simulink model "Disturbance_models"  (R2022a)
settings: Solver=VariableStepAuto  StartTime=0.0  StopTime=10.0  RelTol=1e-3
values from neighbouring files (symbols this model uses):
  A = [0 0 1 0 0 ... (first row only)    [DesignProjectP2.m]    (also in DesignProjectP3.m; DesignProject_OffsetP3.m; mpc_example_regulation.m = [ 	 0,       0,              1,  0, 0; 	 0,       0,        ; mpc_example_tracking.m = [ 	 0,       0,              1,  0, 0; 	 0,       0,        )
  A_dist = [A zeros(5,2) ... (first row only)    [DesignProjectP2.m]
  B = [0;0;0;0;1/La]    [DesignProjectP2.m]    (also in DesignProjectP3.m; DesignProject_OffsetP3.m; mpc_example_regulation.m = [0; 0; 0; 0; 1/La]; mpc_example_tracking.m = [0; 0; 0; 0; 1/La])
  B_dist = [B; zeros(2,1)]    [DesignProjectP2.m]
  C = [1 0 0 0 0 ... (first row only)    [DesignProjectP2.m]    (also in DesignProjectP3.m; DesignProject_OffsetP3.m; mpc_example_regulation.m; mpc_example_tracking.m)
  C_d = [1 0]    [DesignProjectP2.m]    (also in DesignProject_OffsetP3.m)
  C_dist = [0 1 0 0 0 zeros(1,2)]    [DesignProjectP2.m]
  init = [theta_m_init; theta_l_init; thetadot_m_init; thetadot_l_init; Ia_init]    [ELEN90064_Project_Parameters.m]
  K_sin = K_dist(1:5)    [DesignProjectP2.m]    (also in DesignProject_OffsetP3.m = K_dist(7:8))
  Kd_sin = K_dist(6:7)    [DesignProjectP2.m]
  L = place(A', C', observer_poles)'    [DesignProjectP2.m]    (also in DesignProjectP3.m; DesignProject_OffsetP3.m = L_t'; phase2_emc.m = place(A',C',desired_obsv_poles)')
  N_x = G_tf_den(end)/G_tf_num(end)    [DesignProjectP2.m]
  w = 2*pi*1/4    (= 1.57079632679)    [DesignProjectP2.m]    (also in DesignProject_OffsetP3.m)
undefined symbols (not defined in the file or in its folder): J_sin
settings Model: Creator=Admin  LastModifiedBy=Admin

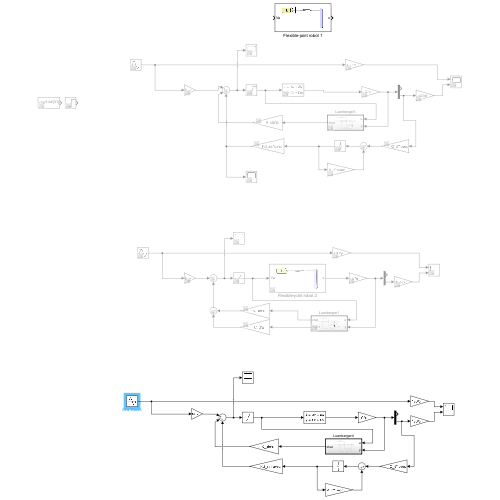
[thumbnail: Simulink's stored preview of the top-level diagram]
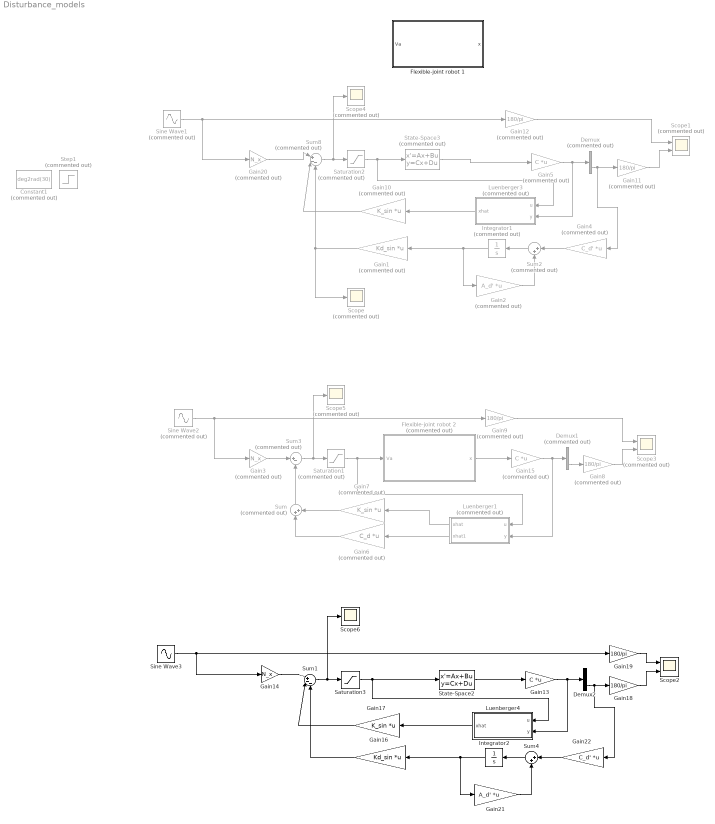
== system Disturbance_models ==
  Constant1 : Constant  Commented=on  Value=deg2rad(30)
  Demux : Demux  Commented=on  Outputs=2
  Demux1 : Demux  Commented=on  Outputs=2
  Demux2 : Demux  Outputs=2
  Flexible-joint robot 1 : Subsystem
      mask Display: image('$imagefile'); % Use "Edit Image" on toolstrip to change.
  Flexible-joint robot 2 : Subsystem  Commented=on
      mask Display: image('$imagefile'); % Use "Edit Image" on toolstrip to change.
  Gain1 : Gain  Commented=on  Gain=Kd_sin  Multiplication=Matrix(K*u) (u vector)
  Gain10 : Gain  Commented=on  Gain=K_sin  Multiplication=Matrix(K*u)
  Gain{8..9,11..12} (4 alike) : Gain  Commented=on  Gain=180/pi
  Gain13 : Gain  Gain=C  Multiplication=Matrix(K*u)
  Gain14 : Gain  Gain=N_x
  Gain15 : Gain  Commented=on  Gain=C  Multiplication=Matrix(K*u)
  Gain16 : Gain  Gain=Kd_sin  Multiplication=Matrix(K*u) (u vector)
  Gain17 : Gain  Gain=K_sin  Multiplication=Matrix(K*u)
  Gain18 : Gain  Gain=180/pi
  Gain19 : Gain  Gain=180/pi
  Gain2 : Gain  Commented=on  Gain=A_d'  Multiplication=Matrix(K*u) (u vector)
  Gain20 : Gain  Commented=on  Gain=N_x
  Gain21 : Gain  Gain=A_d'  Multiplication=Matrix(K*u) (u vector)
  Gain22 : Gain  Gain=C_d'  Multiplication=Matrix(K*u) (u vector)
  Gain3 : Gain  Commented=on  Gain=N_x
  Gain4 : Gain  Commented=on  Gain=C_d'  Multiplication=Matrix(K*u) (u vector)
  Gain5 : Gain  Commented=on  Gain=C  Multiplication=Matrix(K*u)
  Gain6 : Gain  Commented=on  Gain=C_d  Multiplication=Matrix(K*u)
  Gain7 : Gain  Commented=on  Gain=K_sin  Multiplication=Matrix(K*u)
  Integrator1 : Integrator  Commented=on
  Integrator2 : Integrator
  Luenberger1 : Subsystem  Commented=on  TreatAsAtomicUnit=on
  Luenberger3 : Subsystem  Commented=on  TreatAsAtomicUnit=on
  Luenberger4 : Subsystem  TreatAsAtomicUnit=on
  Saturation1 : Saturate  Commented=on  UpperLimit=6  LowerLimit=-6
  Saturation2 : Saturate  Commented=on  UpperLimit=6  LowerLimit=-6
  Saturation3 : Saturate  UpperLimit=6  LowerLimit=-6
  Scope : Scope  Commented=on
  Scope1 : Scope  Commented=on  NumInputPorts=2
  Scope2 : Scope  NumInputPorts=2
  Scope3 : Scope  Commented=on  NumInputPorts=2
  Scope4 : Scope  Commented=on
  Scope5 : Scope  Commented=on
  Scope6 : Scope
  Sine Wave1 : Sin  Commented=on  Amplitude=deg2rad(30)  Frequency=w  Phase=deg2rad(30)  SampleTime=0
  Sine Wave2 : Sin  Commented=on  Amplitude=deg2rad(30)  Frequency=w  Phase=deg2rad(30)  SampleTime=0
  Sine Wave3 : Sin  Amplitude=deg2rad(30)  Frequency=w  Phase=deg2rad(30)  SampleTime=0
  State-Space2 : StateSpace  A=A  B=B  C=eye(5)  D=zeros(5,1)  InitialCondition=0
  State-Space3 : StateSpace  Commented=on  A=A  B=B  C=eye(5)  D=zeros(5,1)  InitialCondition=0
  Step1 : Step  Commented=on  After=deg2rad(60)  SampleTime=0
  Sum : Sum  Commented=on  Inputs=|++
  Sum1 : Sum  Inputs=|+--
  Sum2 : Sum  Commented=on  Inputs=|++
  Sum3 : Sum  Commented=on  Inputs=|+-
  Sum4 : Sum  Inputs=|++
  Sum8 : Sum  Commented=on  Inputs=|+--
  wires:
  Gain20/1 -> Sum8/1
  Gain12/1 -> Scope1/1
  State-Space3/1 -> Gain5/1
  Gain11/1 -> Scope1/2
  Gain10/1 -> Sum8/2
  Sum8/1 -> Scope4/1, Saturation2/1
  Saturation2/1 -> State-Space3/1, Luenberger3/1(u)
  Gain1/1 -> Sum8/3, Scope/1
  Demux/2 -> Gain4/1, Gain11/1
  Sine Wave1/1 -> Gain20/1, Gain12/1
  Gain2/1 -> Sum2/2
  Gain5/1 -> Demux/1, Luenberger3/2(y)
  Sum2/1 -> Integrator1/1
  Integrator1/1 -> Gain1/1, Gain2/1
  Gain4/1 -> Sum2/1
  Gain15/1 -> Demux1/1, Luenberger1/2(y)
  Sine Wave2/1 -> Gain9/1, Gain3/1
  Demux1/2 -> Gain8/1
  Luenberger1/1(xhat) -> Gain7/1
  Saturation1/1 -> Flexible-joint robot 2/1(Va), Luenberger1/1(u)
  Sum3/1 -> Saturation1/1, Scope5/1
  Gain7/1 -> Sum/2
  Gain8/1 -> Scope3/2
  Flexible-joint robot 2/1(x) -> Gain15/1
  Gain9/1 -> Scope3/1
  Gain3/1 -> Sum3/1
  Luenberger1/2(xhat1) -> Gain6/1
  Gain6/1 -> Sum/1
  Gain16/1 -> Sum1/3
  Gain14/1 -> Sum1/1
  Gain19/1 -> Scope2/1
  State-Space2/1 -> Gain13/1
  Gain18/1 -> Scope2/2
  Gain17/1 -> Sum1/2
  Sum1/1 -> Scope6/1, Saturation3/1
  Saturation3/1 -> Luenberger4/1(u), State-Space2/1
  Luenberger4/1(xhat) -> Gain17/1
  Sine Wave3/1 -> Gain19/1, Gain14/1
  Gain13/1 -> Luenberger4/2(y), Demux2/1
  Sum/1 -> Sum3/2
  Luenberger3/1(xhat) -> Gain10/1
  Sum4/1 -> Integrator2/1
  Gain21/1 -> Sum4/2
  Gain22/1 -> Sum4/1
  Integrator2/1 -> Gain16/1, Gain21/1
  Demux2/2 -> Gain22/1, Gain18/1

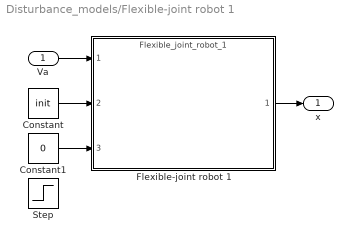
== system Disturbance_models/Flexible-joint robot 1 ==
  Va : Inport
  Constant : Constant  Value=init
  Constant1 : Constant  Value=0
  Flexible-joint robot 1 : ModelReference  ModelNameDialog=Flexible_joint_robot_1  ModelReferenceVersion=1.65  CopyOfModelProtected=on
  Step : Step  After=0.05  SampleTime=0
  x : Outport
  wires:
  Constant/1 -> Flexible-joint robot 1/2
  Flexible-joint robot 1/1 -> x/1
  Va/1 -> Flexible-joint robot 1/1
  Constant1/1 -> Flexible-joint robot 1/3

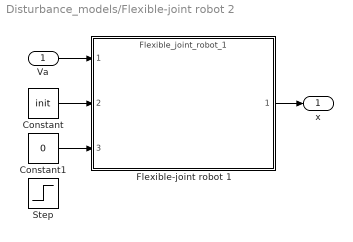
== system Disturbance_models/Flexible-joint robot 2 ==
  Va : Inport
  Constant : Constant  Value=init
  Constant1 : Constant  Value=0
  Flexible-joint robot 1 : ModelReference  ModelNameDialog=Flexible_joint_robot_1  ModelReferenceVersion=1.65  CopyOfModelProtected=on
  Step : Step  After=0.05  SampleTime=0
  x : Outport
  wires:
  Constant1/1 -> Flexible-joint robot 1/3
  Va/1 -> Flexible-joint robot 1/1
  Flexible-joint robot 1/1 -> x/1
  Constant/1 -> Flexible-joint robot 1/2

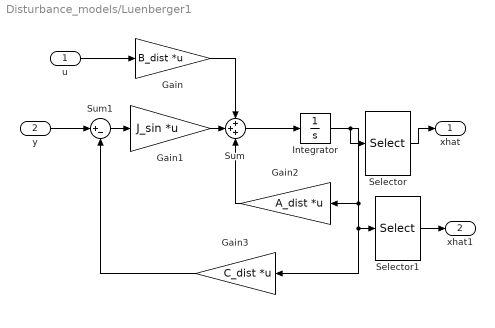
== system Disturbance_models/Luenberger1 ==
  u : Inport
  y : Inport  Port=2
  Gain : Gain  Gain=B_dist  Multiplication=Matrix(K*u) (u vector)
  Gain1 : Gain  Gain=J_sin  Multiplication=Matrix(K*u) (u vector)
  Gain2 : Gain  Gain=A_dist  Multiplication=Matrix(K*u) (u vector)
  Gain3 : Gain  Gain=C_dist  Multiplication=Matrix(K*u) (u vector)
  Integrator : Integrator
  Selector : Selector  InputPortWidth=7  IndexOptions=Index vector (dialog)  Indices=[1 2 3 4 5]  OutputSizes=1
  Selector1 : Selector  InputPortWidth=7  IndexOptions=Index vector (dialog)  Indices=[6 7]  OutputSizes=1
  Sum : Sum  Inputs=+++
  Sum1 : Sum  Inputs=|+-
  xhat : Outport
  xhat1 : Outport  Port=2
  wires:
  u/1 -> Gain/1
  Gain/1 -> Sum/1
  y/1 -> Sum1/1
  Sum1/1 -> Gain1/1
  Gain1/1 -> Sum/2
  Sum/1 -> Integrator/1
  Integrator/1 -> Selector1/1, Gain3/1, Gain2/1, Selector/1
  Gain2/1 -> Sum/3
  Gain3/1 -> Sum1/2
  Selector/1 -> xhat/1
  Selector1/1 -> xhat1/1

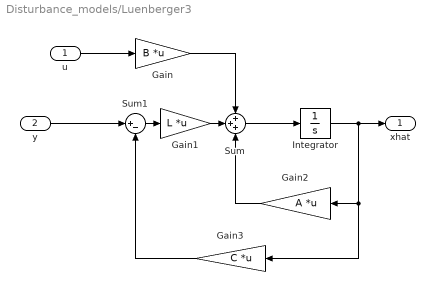
== system Disturbance_models/Luenberger3 ==
  u : Inport
  y : Inport  Port=2
  Gain : Gain  Gain=B  Multiplication=Matrix(K*u) (u vector)
  Gain1 : Gain  Gain=L  Multiplication=Matrix(K*u) (u vector)
  Gain2 : Gain  Gain=A  Multiplication=Matrix(K*u) (u vector)
  Gain3 : Gain  Gain=C  Multiplication=Matrix(K*u) (u vector)
  Integrator : Integrator
  Sum : Sum  Inputs=+++
  Sum1 : Sum  Inputs=|+-
  xhat : Outport
  wires:
  Gain3/1 -> Sum1/2
  Gain2/1 -> Sum/3
  Integrator/1 -> xhat/1, Gain2/1, Gain3/1
  Sum/1 -> Integrator/1
  Gain1/1 -> Sum/2
  Sum1/1 -> Gain1/1
  y/1 -> Sum1/1
  Gain/1 -> Sum/1
  u/1 -> Gain/1

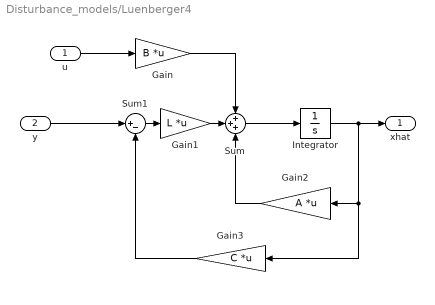
== system Disturbance_models/Luenberger4 ==
  u : Inport
  y : Inport  Port=2
  Gain : Gain  Gain=B  Multiplication=Matrix(K*u) (u vector)
  Gain1 : Gain  Gain=L  Multiplication=Matrix(K*u) (u vector)
  Gain2 : Gain  Gain=A  Multiplication=Matrix(K*u) (u vector)
  Gain3 : Gain  Gain=C  Multiplication=Matrix(K*u) (u vector)
  Integrator : Integrator
  Sum : Sum  Inputs=+++
  Sum1 : Sum  Inputs=|+-
  xhat : Outport
  wires:
  u/1 -> Gain/1
  Gain/1 -> Sum/1
  y/1 -> Sum1/1
  Sum1/1 -> Gain1/1
  Gain1/1 -> Sum/2
  Sum/1 -> Integrator/1
  Integrator/1 -> Gain3/1, Gain2/1, xhat/1
  Gain2/1 -> Sum/3
  Gain3/1 -> Sum1/2
